simulink model "Signal_Builder_To_Workspace_LONG"  (R2014a)
settings: Solver=ode45  StartTime=0.0  StopTime=5  RelTol=1e-3
PostLoadFcn:
  | warning off Simulink:Engine:UsingDefaultMaxStepSize
  | warning off Simulink:Engine:UsingDiscreteSolver
undefined symbols (not defined in the file or in its folder): sigbuilder_block
Description:
  | Copyright 2014 The MathWorks, Inc.
settings Model: Creator=smiller  LastModifiedBy=psanghvi
settings DebuggingCC: UnderspecifiedInitializationDetection=Classic  StateNameClashWarn=warning

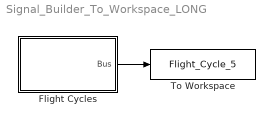
== system Signal_Builder_To_Workspace_LONG ==
  Flight Cycles : Subsystem  Tag=STV Subsys  LoadFcn=sigbuilder_block('load');  StartFcn=sigbuilder_block('start');  StopFcn=sigbuilder_block('stop');  ClipboardFcn=sigbuilder_block('clipboard');  mask(Sigbuilder block){}
      mask help: Simulink:masks:SigbuilderBlock_MD
      mask init:
      | if ~strcmp(get_param(bdroot(gcbh),'SimulationStatus'),'stopped') tuvar = sigbuilder_block('maskInit'); end
      settings: CopyFcn=sigbuilder_block('copy');  DeleteFcn=sigbuilder_block('delete');  ModelCloseFcn=sigbuilder_block('modelClose');  PreSaveFcn=sigbuilder_block('preSave');  PauseFcn=sigbuilder_block('pause');  ContinueFcn=sigbuilder_block('continue');  NameChangeFcn=sigbuilder_block('namechange');  OpenFcn=sigbuilder_block('open',[24.2069 76.3448 906.207 605.793 ]);  CloseFcn=sigbuilder_block('close');
      mask Display: plot(0, 0, 100, 100,[2, 2, 32, 32, 2], [68, 8, 8, 68, 68],[32, 2], [38, 38], [32, 19, 2],[53, 60, 44], [32, 17, 17, 2],[16, 16, 31, 31]);txt = getActiveGroup(gcbh);text(2, 100, txt,'verticalAlignment', 'top');
  To Workspace : ToWorkspace  VariableName=Flight_Cycle_5  SaveFormat=Structure With Time  SampleTime=-1
  wires:
  Flight Cycles/1(Bus) -> To Workspace/1

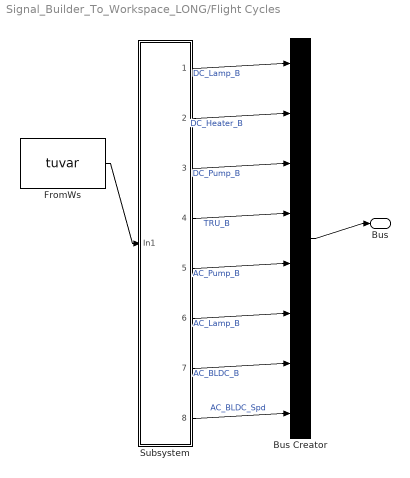
== system Signal_Builder_To_Workspace_LONG/Flight Cycles ==
  Bus Creator : BusCreator  Tag=Bus Creator  Inputs=8
  FromWs : FromWorkspace  Tag=STV FromWs  VariableName=tuvar  SampleTime=0
      SigBuilderData=|
      | common.afterFinalStr = 'Extrapolate'
      | common.sampleTime = '0'
      | dataSet(1).timeRange = [0 10]
      | dataSet(1).name = 'All On'
      | dataSet(2).timeRange = [0 400]
      | dataSet(2).name = 'Cycle 1'
      | dataSet(3).timeRange = [0 10]
      | dataSet(3).name = 'Cycle 2'
      | dataSet(4).timeRange = [0 10]
      | dataSet(4).name = 'Cycle 3'
      | dataSet(5).timeRange = [0 10]
      | dataSet(5).name = 'Lamp_Test'
      | sbobj.Groups(1).Name = 'All On'
      | sbobj.Groups(1).Signals(1).Name = 'DC_Lamp_B'
      | sbobj.Groups(1).Signals(1).XData = [0 5 10]
      | sbobj.Groups(1).Signals(1).YData = [1 1 1]
      | sbobj.Groups(1).Signals(2).Name = 'DC_Heater_B'
      | sbobj.Groups(1).Signals(2).XData = [0 5 10]
      | sbobj.Groups(1).Signals(2).YData = [1 1 1]
      | sbobj.Groups(1).Signals(3).Name = 'DC_Pump_B'
      | sbobj.Groups(1).Signals(3).XData = [0 5 10]
      | sbobj.Groups(1).Signals(3).YData = [1 1 1]
      | sbobj.Groups(1).Signals(4).Name = 'TRU_B'
      | sbobj.Groups(1).Signals(4).XData = [0 5 10]
      | sbobj.Groups(1).Signals(4).YData = [1 1 1]
      | sbobj.Groups(1).Signals(5).Name = 'AC_Pump_B'
      | sbobj.Groups(1).Signals(5).XData = [0 5 10]
      | sbobj.Groups(1).Signals(5).YData = [1 1 1]
      | sbobj.Groups(1).Signals(6).Name = 'AC_Lamp_B'
      | sbobj.Groups(1).Signals(6).XData = [0 5 10]
      | sbobj.Groups(1).Signals(6).YData = [1 1 1]
      | sbobj.Groups(1).Signals(7).Name = 'AC_BLDC_B'
      | sbobj.Groups(1).Signals(7).XData = [0 4 10]
      | sbobj.Groups(1).Signals(7).YData = [500 500 500]
      | sbobj.Groups(1).Signals(8).Name = 'AC_BLDC_Spd'
      | sbobj.Groups(1).Signals(8).XData = [0 1 10]
      | sbobj.Groups(1).Signals(8).YData = [0 0 0]
      | sbobj.Groups(2).Name = 'Cycle 1'
      | sbobj.Groups(2).Signals(1).Name = 'DC_Lamp_B'
      | sbobj.Groups(2).Signals(1).XData = [0 0.5 0.5 1.5 1.5 3 3 400]
      | sbobj.Groups(2).Signals(1).YData = [1 1 0 0 1 1 0 0]
      | sbobj.Groups(2).Signals(2).Name = 'DC_Heater_B'
      | sbobj.Groups(2).Signals(2).XData = [0 1 1 2.5 2.5 3.5 3.5 400]
      | sbobj.Groups(2).Signals(2).YData = [1 1 0 0 1 1 0 0]
      | sbobj.Groups(2).Signals(3).Name = 'DC_Pump_B'
      | sbobj.Groups(2).Signals(3).XData = [0 2 2 3.56 4 400]
      | sbobj.Groups(2).Signals(3).YData = [1 1 0 0 0 0]
      | sbobj.Groups(2).Signals(4).Name = 'TRU_B'
      | sbobj.Groups(2).Signals(4).XData = [0 5 400]
      | sbobj.Groups(2).Signals(4).YData = [1 1 1]
      | sbobj.Groups(2).Signals(5).Name = 'AC_Pump_B'
      | sbobj.Groups(2).Signals(5).XData = [0 5 400]
      | sbobj.Groups(2).Signals(5).YData = [1 1 1]
      | sbobj.Groups(2).Signals(6).Name = 'AC_Lamp_B'
      | sbobj.Groups(2).Signals(6).XData = [0 5 400]
      | sbobj.Groups(2).Signals(6).YData = [1 1 1]
      | sbobj.Groups(2).Signals(7).Name = 'AC_BLDC_B'
      | sbobj.Groups(2).Signals(7).XData = [0 5 400]
      | sbobj.Groups(2).Signals(7).YData = [1 1 1]
      | sbobj.Groups(2).Signals(8).Name = 'AC_BLDC_Spd'
      | sbobj.Groups(2).Signals(8).XData = [0 5 400]
      | sbobj.Groups(2).Signals(8).YData = [0 0 0]
      | sbobj.Groups(2).TimeRange = [0 400]
      | sbobj.Groups(3).Name = 'Cycle 2'
      | sbobj.Groups(3).Signals(1).Name = 'DC_Lamp_B'
      | sbobj.Groups(3).Signals(1).XData = [0 1 1 3 3 4 4 10]
      | sbobj.Groups(3).Signals(1).YData = [1 1 0 0 1 1 0 0]
      | sbobj.Groups(3).Signals(2).Name = 'DC_Heater_B'
      | sbobj.Groups(3).Signals(2).XData = [0 1 1 3 3 4 4 10]
      | sbobj.Groups(3).Signals(2).YData = [1 1 0 0 1 1 -0.02 -0.02]
      | sbobj.Groups(3).Signals(3).Name = 'DC_Pump_B'
      | sbobj.Groups(3).Signals(3).XData = [0 2 3.56 4 10]
      | sbobj.Groups(3).Signals(3).YData = [1 1 1 1 1]
      | sbobj.Groups(3).Signals(4).Name = 'TRU_B'
      | sbobj.Groups(3).Signals(4).XData = [0 5 10]
      | sbobj.Groups(3).Signals(4).YData = [1 1 1]
      | sbobj.Groups(3).Signals(5).Name = 'AC_Pump_B'
      | sbobj.Groups(3).Signals(5).XData = [0 5 10]
      | sbobj.Groups(3).Signals(5).YData = [1 1 1]
      | sbobj.Groups(3).Signals(6).Name = 'AC_Lamp_B'
      | sbobj.Groups(3).Signals(6).XData = [0 1 1 3 3 4 4 10]
      | sbobj.Groups(3).Signals(6).YData = [1 1 0 0 1 1 0 0]
      | sbobj.Groups(3).Signals(7).Name = 'AC_BLDC_B'
      | sbobj.Groups(3).Signals(7).XData = [0 5 10]
      | sbobj.Groups(3).Signals(7).YData = [1 1 1]
      | sbobj.Groups(3).Signals(8).Name = 'AC_BLDC_Spd'
      | sbobj.Groups(3).Signals(8).XData = [0 1.4 1.4 1.9 1.9 2.4 2.4 3 3 10]
      | sbobj.Groups(3).Signals(8).YData = [0 0 500 500 0 0 -500 -500 0 0]
      | sbobj.Groups(4).Name = 'Cycle 3'
      | sbobj.Groups(4).Signals(1).Name = 'DC_Lamp_B'
      | sbobj.Groups(4).Signals(1).XData = [0 1 1 3 3 4 4 10]
      | sbobj.Groups(4).Signals(1).YData = [1 1 0 0 1 1 0 0]
      | sbobj.Groups(4).Signals(2).Name = 'DC_Heater_B'
      | sbobj.Groups(4).Signals(2).XData = [0 1 1 2 2 3.63 3.63 10]
      | sbobj.Groups(4).Signals(2).YData = [1 1 0 0 1 1 -0.02 -0.02]
      | sbobj.Groups(4).Signals(3).Name = 'DC_Pump_B'
      | sbobj.Groups(4).Signals(3).XData = [0 2 3.56 4 10]
      | sbobj.Groups(4).Signals(3).YData = [1 1 1 1 1]
      | sbobj.Groups(4).Signals(4).Name = 'TRU_B'
      | sbobj.Groups(4).Signals(4).XData = [0 5 10]
      | sbobj.Groups(4).Signals(4).YData = [1 1 1]
      | sbobj.Groups(4).Signals(5).Name = 'AC_Pump_B'
      | sbobj.Groups(4).Signals(5).XData = [0 5 10]
      | sbobj.Groups(4).Signals(5).YData = [1 1 1]
      | sbobj.Groups(4).Signals(6).Name = 'AC_Lamp_B'
      | sbobj.Groups(4).Signals(6).XData = [0 1 1 1.71 1.71 2.53 2.53 10]
      | sbobj.Groups(4).Signals(6).YData = [1 1 0 0 1 1 0 0]
      | sbobj.Groups(4).Signals(7).Name = 'AC_BLDC_B'
      | sbobj.Groups(4).Signals(7).XData = [0 5 10]
      | sbobj.Groups(4).Signals(7).YData = [1 1 1]
      | sbobj.Groups(4).Signals(8).Name = 'AC_BLDC_Spd'
      | sbobj.Groups(4).Signals(8).XData = [0 0.77 0.77 1.9 1.9 2.4 2.4 3.61 3.61 10]
      | sbobj.Groups(4).Signals(8).YData = [0 0 500 500 0 0 -500 -500 0 0]
      | sbobj.Groups(5).Name = 'Lamp_Test'
      | sbobj.Groups(5).Signals(1).Name = 'DC_Lamp_B'
      | sbobj.Groups(5).Signals(1).XData = [0 5 10]
      | sbobj.Groups(5).Signals(1).YData = [1 1 1]
      | sbobj.Groups(5).Signals(2).Name = 'DC_Heater_B'
      | sbobj.Groups(5).Signals(2).XData = [0 5 10]
      | sbobj.Groups(5).Signals(2).YData = [1 1 1]
      | sbobj.Groups(5).Signals(3).Name = 'DC_Pump_B'
      | sbobj.Groups(5).Signals(3).XData = [0 5 10]
      | sbobj.Groups(5).Signals(3).YData = [1 1 1]
      | sbobj.Groups(5).Signals(4).Name = 'TRU_B'
      | sbobj.Groups(5).Signals(4).XData = [0 5 10]
      | sbobj.Groups(5).Signals(4).YData = [1 1 1]
      | sbobj.Groups(5).Signals(5).Name = 'AC_Pump_B'
      | sbobj.Groups(5).Signals(5).XData = [0 5 10]
      | sbobj.Groups(5).Signals(5).YData = [1 1 1]
      | sbobj.Groups(5).Signals(6).Name = 'AC_Lamp_B'
      | sbobj.Groups(5).Signals(6).XData = [0 2 2 3 3 4 4 5 5 10]
      | sbobj.Groups(5).Signals(6).YData = [1 1 0 0 1 1 0 0 1 1]
      | sbobj.Groups(5).Signals(7).Name = 'AC_BLDC_B'
      | sbobj.Groups(5).Signals(7).XData = [0 4 10]
      | sbobj.Groups(5).Signals(7).YData = [500 500 500]
      | sbobj.Groups(5).Signals(8).Name = 'AC_BLDC_Spd'
      | sbobj.Groups(5).Signals(8).XData = [0 10]
      | sbobj.Groups(5).Signals(8).YData = [0 0]
  Subsystem : Subsystem
  Bus : Outport
  wires:
  FromWs/1 -> Subsystem/1(In1)
  Subsystem/1(DC_Lamp_B) -> Bus Creator/1  "DC_Lamp_B"
  Subsystem/2(DC_Heater_B) -> Bus Creator/2  "DC_Heater_B"
  Subsystem/3(DC_Pump_B) -> Bus Creator/3  "DC_Pump_B"
  Subsystem/4(TRU_B) -> Bus Creator/4  "TRU_B"
  Subsystem/5(AC_Pump_B) -> Bus Creator/5  "AC_Pump_B"
  Subsystem/6(AC_Lamp_B) -> Bus Creator/6  "AC_Lamp_B"
  Subsystem/7(AC_BLDC_B) -> Bus Creator/7  "AC_BLDC_B"
  Subsystem/8(AC_BLDC_Spd) -> Bus Creator/8  "AC_BLDC_Spd"
  Bus Creator/1 -> Bus/1

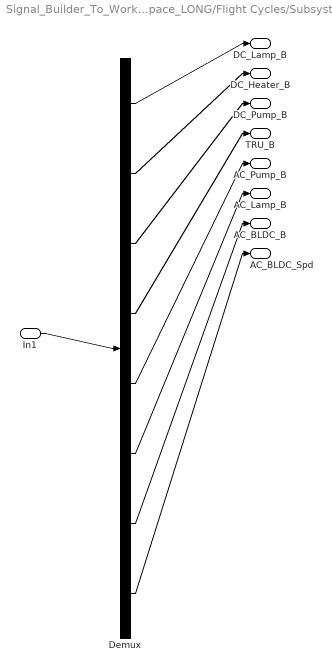
== system Signal_Builder_To_Workspace_LONG/Flight Cycles/Subsystem ==
  In1 : Inport
  Demux : Demux  Tag=STV Demux  Outputs=8
  DC_Lamp_B : Outport  Tag=STV Outport
  DC_Heater_B : Outport  Tag=STV Outport  Port=2
  DC_Pump_B : Outport  Tag=STV Outport  Port=3
  TRU_B : Outport  Tag=STV Outport  Port=4
  AC_Pump_B : Outport  Tag=STV Outport  Port=5
  AC_Lamp_B : Outport  Tag=STV Outport  Port=6
  AC_BLDC_B : Outport  Tag=STV Outport  Port=7
  AC_BLDC_Spd : Outport  Tag=STV Outport  Port=8
  wires:
  Demux/1 -> DC_Lamp_B/1
  Demux/2 -> DC_Heater_B/1
  Demux/3 -> DC_Pump_B/1
  Demux/4 -> TRU_B/1
  Demux/5 -> AC_Pump_B/1
  Demux/6 -> AC_Lamp_B/1
  Demux/7 -> AC_BLDC_B/1
  Demux/8 -> AC_BLDC_Spd/1
  In1/1 -> Demux/1
